simulink model "input"  (R2021a)
settings: Solver=FixedStepAuto  StartTime=0.0  StopTime=10.0  RelTol=1e-3
settings Model: Creator=k39win3  LastModifiedBy=k39win3

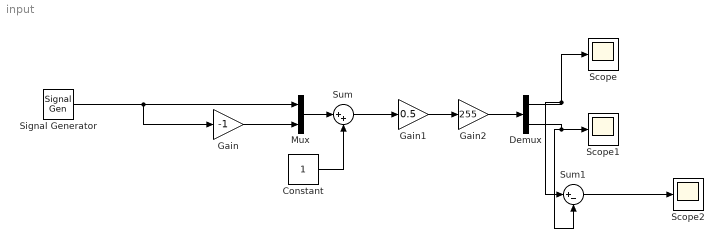
== system input ==
  Constant : Constant
  Demux : Demux  Outputs=2
  Gain : Gain  Gain=-1
  Gain1 : Gain  Gain=0.5
  Gain2 : Gain  Gain=255
  Mux : Mux  Inputs=2
  Scope : Scope
  Scope1 : Scope
  Scope2 : Scope
  Signal Generator : SignalGenerator  WaveForm=sawtooth  Units=rad/sec
  Sum : Sum  Inputs=|++
  Sum1 : Sum  Inputs=|+-
  wires:
  Demux/1 -> Scope/1, Sum1/1
  Signal Generator/1 -> Gain/1, Mux/1
  Mux/1 -> Sum/1
  Gain2/1 -> Demux/1
  Constant/1 -> Sum/2
  Gain/1 -> Mux/2
  Demux/2 -> Scope1/1, Sum1/2
  Sum/1 -> Gain1/1
  Gain1/1 -> Gain2/1
  Sum1/1 -> Scope2/1
